simulink model "RobotX_TrajectoryPlanning"  (R2024a)
settings: Solver=ode45  StartTime=0.0  StopTime=17.77  MaxStep=1e-3  MinStep=1e-5  RelTol=1e-3
libraries: matrix_library x2, dspinverses x1, RobotX_Lib x1
settings Model: Creator=margaridaestrela  LastModifiedBy=margaridaestrela
settings SolverCC: MaxConsecutiveMinStep=100  ZeroCrossControl=DisableAll
settings DebuggingCC: SignalInfNanChecking=error

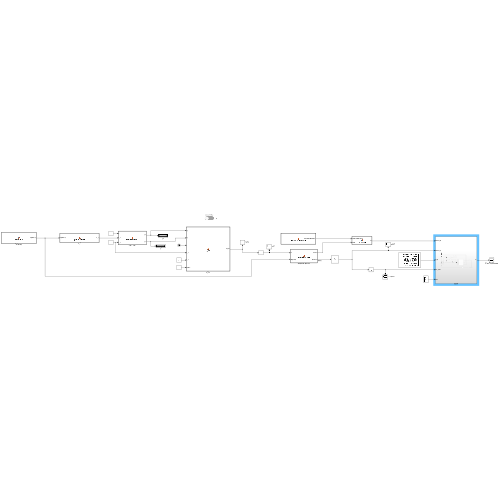
[thumbnail: Simulink's stored preview of the top-level diagram]
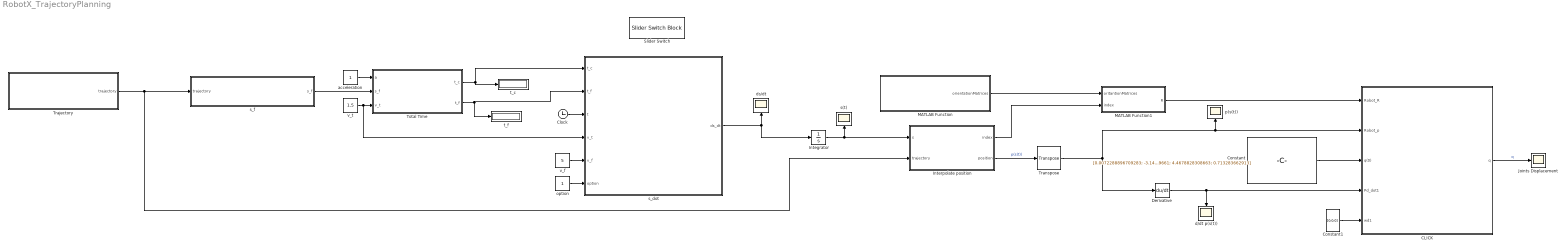
== system RobotX_TrajectoryPlanning ==
  CLICK : Subsystem
  Clock : Clock
  Constant : Constant  Value=[0.0072288896709283; -3.1404691212397; -57.815493873629; 68.626124143896; -3.1193903419661; 4.4678828308663; 0.713283662913]  VectorParams1D=off
  Constant1 : Constant  Value=[0;0;0]  VectorParams1D=off
  Derivative : Derivative
  Integrator : Integrator
  Interpolate position : MATLAB Function  TreatAsAtomicUnit=on
  Joints Displacement : Scope
  MATLAB Function : MATLAB Function  TreatAsAtomicUnit=on
  MATLAB Function1 : MATLAB Function  TreatAsAtomicUnit=on
  Slider Switch : SliderSwitchBlock
      settings: Values={{'1', '2'}, [1 2]}
  Total Time : MATLAB Function  TreatAsAtomicUnit=on
  Trajectory : MATLAB Function  TreatAsAtomicUnit=on
  Transpose : matrix_library/Transpose
  acceleration : Constant
  d/dt p(s(t)) : Scope
  ds/dt : Scope
  option : Constant
  p(s(t)) : Scope
  s(t) : Scope
  s_dot : MATLAB Function  TreatAsAtomicUnit=on
  s_f : MATLAB Function  TreatAsAtomicUnit=on
  t_c : Display
  t_f : Display
  v_f : Constant  Value=5
  v_t : Constant  Value=1.5
  wires:
  acceleration/1 -> Total Time/1(a)
  s_f/1(s_f) -> Total Time/2(s_f)
  Derivative/1 -> CLICK/4(Pd_dot1), d/dt p(s(t))/1
  v_t/1 -> s_dot/4(v_t), Total Time/3(v_t)
  Interpolate position/2(position) -> Transpose/1  "p(s(t))"
  Integrator/1 -> Interpolate position/1(s), s(t)/1
  s_dot/1(ds_dt) -> ds/dt/1, Integrator/1
  Total Time/1(t_c) -> s_dot/1(t_c), t_c/1
  Total Time/2(t_f) -> s_dot/2(t_f), t_f/1
  Trajectory/1(trajectory) -> Interpolate position/2(trajectory), s_f/1(trajectory)
  v_f/1 -> s_dot/5(v_f)
  option/1 -> s_dot/6(option)
  Transpose/1 -> Derivative/1, CLICK/2(Robot_p), p(s(t))/1
  Clock/1 -> s_dot/3(t)
  Constant/1 -> CLICK/3(q(0))
  MATLAB Function/1(orientationMatrices) -> MATLAB Function1/1(oritantionMatrices)
  Interpolate position/1(index) -> MATLAB Function1/2(index)
  Constant1/1 -> CLICK/5(wd1)
  MATLAB Function1/1(R) -> CLICK/1(Robot_R)
  CLICK/1(q) -> Joints Displacement/1  "q"

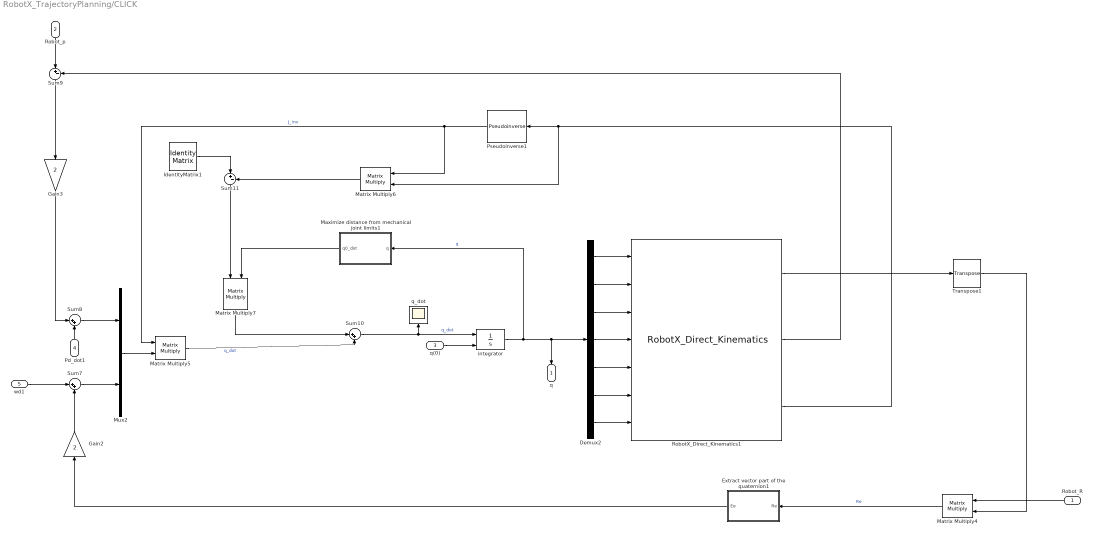
== system RobotX_TrajectoryPlanning/CLICK ==
  Robot_R : Inport
  Robot_p : Inport  Port=2
  q(0) : Inport  Port=3
  Pd_dot1 : Inport  Port=4
  wd1 : Inport  Port=5
  Demux2 : Demux  Outputs=7
  Extract vector part of the quaternion1 : MATLAB Function  TreatAsAtomicUnit=on
  Gain2 : Gain  Gain=2
  Gain3 : Gain  Gain=2
  IdentityMatrix1 : IdentityMatrix  OutputDimensions=7
  Matrix Multiply{4..7} (4 alike) : Product  Multiplication=Matrix(*)
  Maximize distance from mechanical joint limits1 : MATLAB Function  TreatAsAtomicUnit=on
  Mux2 : Mux  Inputs=2
  Pseudoinverse1 : dspinverses/Pseudoinverse  wanterr=off  SimulateUsing=Interpreted execution
  RobotX_Direct_Kinematics1 : RobotX_Lib/RobotX_Direct_Kinematics  SystemSampleTime=-1  VariantActivationTime=update diagram  AllowFlexibleInterface=on  Latency=0  AutoFrameSizeCalculation=off
  Sum10 : Sum  Inputs=|++
  Sum11 : Sum  Inputs=|+-
  Sum7 : Sum  Inputs=|++
  Sum8 : Sum  Inputs=|++
  Sum9 : Sum  Inputs=|+-
  Transpose1 : matrix_library/Transpose
  integrator : Integrator  InitialConditionSource=external
  q_dot : Scope
  q : Outport
  wires:
  Sum9/1 -> Gain3/1
  Matrix Multiply4/1 -> Extract vector part of the quaternion1/1(Re)  "Re"
  Matrix Multiply5/1 -> Sum10/2  "q_dot"
  Sum8/1 -> Mux2/1
  Robot_R/1 -> Matrix Multiply4/1
  Gain3/1 -> Sum8/1
  RobotX_Direct_Kinematics1/1 -> Transpose1/1
  integrator/1 -> q/1, Demux2/1, Maximize distance from mechanical joint limits1/1(q)  "q"
  Demux2/7 -> RobotX_Direct_Kinematics1/7
  RobotX_Direct_Kinematics1/3 -> Matrix Multiply6/2, Pseudoinverse1/1
  Maximize distance from mechanical joint limits1/1(q0_dot) -> Matrix Multiply7/2
  q(0)/1 -> integrator/2
  Gain2/1 -> Sum7/2
  Demux2/3 -> RobotX_Direct_Kinematics1/3
  Sum11/1 -> Matrix Multiply7/1
  Matrix Multiply6/1 -> Sum11/2
  Transpose1/1 -> Matrix Multiply4/2
  Demux2/4 -> RobotX_Direct_Kinematics1/4
  Demux2/5 -> RobotX_Direct_Kinematics1/5
  Demux2/6 -> RobotX_Direct_Kinematics1/6
  Pseudoinverse1/1 -> Matrix Multiply5/1, Matrix Multiply6/1  "J_inv"
  IdentityMatrix1/1 -> Sum11/1
  Mux2/1 -> Matrix Multiply5/2
  Robot_p/1 -> Sum9/1
  Sum7/1 -> Mux2/2
  Demux2/2 -> RobotX_Direct_Kinematics1/2
  Extract vector part of the quaternion1/1(Ee) -> Gain2/1
  Sum10/1 -> integrator/1, q_dot/1  "q_dot"
  RobotX_Direct_Kinematics1/2 -> Sum9/2
  Matrix Multiply7/1 -> Sum10/1
  Demux2/1 -> RobotX_Direct_Kinematics1/1
  wd1/1 -> Sum7/1
  Pd_dot1/1 -> Sum8/2

== matlab function RobotX_TrajectoryPlanning/Interpolate position ==
  data: index output; s input; trajectory input; position output
function [index, position] = interpolatePosition(s, trajectory)
    % Ensure s is within the bounds of cumulative distance
    cumulativeDistance = computeCumulativeDistance(trajectory);
    %s = min(max(s, cumulativeDistance(1)), cumulativeDistance(end));
    
    % Interpolate position
    position = interp1(cumulativeDistance, trajectory, s, 'linear', 'extrap');

    % Find the nearest index in the cumulative distance array
    [~, index] = min(abs(cumulativeDistance - s));
end

function cumulativeDistance = computeCumulativeDistance(trajectory)
    % Calculate distances between consecutive points
    distances = sqrt(sum(diff(trajectory).^2, 2));

    % Replace zeros with a small value (epsilon)
    eps = 1e-3;
    distances(distances == 0) = eps;
    
    % Calculate cumulative distance
    cumulativeDistance = [0; cumsum(distances)];
    
    % Ensure cumulativeDistance is strictly increasing by a minimum
    % difference of epsilon
    for i = 2:length(cumulativeDistance)
        while cumulativeDistance(i) <= cumulativeDistance(i-1) + eps;
            cumulativeDistance(i) = cumulativeDistance(i) + eps;
        end
    end
end

== matlab function RobotX_TrajectoryPlanning/CLICK/Extract vector part of the quaternion1 ==
  data: Re input; Ee output
function Ee = fcn(Re)
    % Initialize the output vector
    Ee = zeros(3, 1);

    % Compute the angle theta
    cos_theta = (Re(1,1) + Re(2,2) + Re(3,3) - 1) / 2;

    if cos_theta < -1 || cos_theta > 1
        return
    end

    theta = acos(cos_theta);

    % Initialize rx, ry, rz
    rx = 0;
    ry = 0;
    rz = 0;

    % Check for singularity at theta = 0 or theta = pi
    if sin(theta) == 0
        % Handle the case when theta is 0 or pi
        if cos_theta == 1
            % When theta is 0
            Ee = [0; 0; 0];
        else
            % When theta is pi
            % Choose the largest diagonal element for numerical stability
            [~, max_index] = max([Re(1,1), Re(2,2), Re(3,3)]);
            switch max_index
                case 1
                    rx = sqrt((Re(1,1) + 1) / 2);
                    ry = Re(2,1) / (2 * rx);
                    rz = Re(3,1) / (2 * rx);
                case 2
                    ry = sqrt((Re(2,2) + 1) / 2);
                    rx = Re(1,2) / (2 * ry);
                    rz = Re(3,2) / (2 * ry);
                case 3
                    rz = sqrt((Re(3,3) + 1) / 2);
                    rx = Re(1,3) / (2 * rz);
                    ry = Re(2,3) / (2 * rz);
            end
            Ee = [rx; ry; rz];
        end
    else
        % Compute the vector part for theta in (0, pi)
        rx = Re(3, 2) - Re(2, 3);
        ry = Re(1, 3) - Re(3, 1);
        rz = Re(2, 1) - Re(1, 2);
        Ee = (1 / (2 * sin(theta))) * [rx; ry; rz];
    end
end

== matlab function RobotX_TrajectoryPlanning/MATLAB Function ==
  data: orientationMatrices output
function orientationMatrices = loadOrientationMatrices
    data = load('orientationMatrices.mat');
    orientationMatrices = data.orientationMatrices;
end

== matlab function RobotX_TrajectoryPlanning/Trajectory ==
  data: trajectory output
function trajectory = loadTrajectory()
    data = load('trajectoryData.mat');
    trajectory = data.trajectory;
end

== matlab function RobotX_TrajectoryPlanning/s_f ==
  data: trajectory input; s_f output
function s_f = getTotalDistance(trajectory)
    distances = sqrt(sum(diff(trajectory).^2, 2));
    s_f = sum(distances);
end

== matlab function RobotX_TrajectoryPlanning/Total Time ==
  data: a input; s_f input; v_t input; t_c output; t_f output
function [t_c, t_f] = calculateTotalTime(a, s_f, v_t)
    % Calculate time to reach maximum velocity (acceleration phase)
    t_c = v_t / a;
    
    % Calculate distance covered during acceleration (and deceleration)
    d_c = 1/2 * a * t_c^2;
    
    % Calculate distance covered at constant velocity
    d_const = s_f - 2 * d_c;
    
    % Check if the distance for acceleration and deceleration is feasible
    if d_c * 2 > s_f
        error('Total distance is too short for the given acceleration and maximum velocity.');
    end
    
    % Calculate time for constant velocity phase
    t_const = d_const / v_t;
    
    % Total time of the trajectory
    t_f = t_c + t_const + t_c; % t_c is used for both acceleration and deceleration phases
end

== matlab function RobotX_TrajectoryPlanning/CLICK/Maximize distance from mechanical joint limits1 ==
  data: q0_dot output; q input
function q0_dot = fcn(q)
    n = length(q);  % Number of elements in q

    q_max = [350; deg2rad(170); deg2rad(45); deg2rad(156); deg2rad(185); deg2rad(120); deg2rad(350)];
    q_min = [-350; deg2rad(-170); deg2rad(-190); deg2rad(-120); deg2rad(-185); deg2rad(-120); deg2rad(-350)];

    q_dif = q_max - q_min;

    % Manually derive the differentiation
    w_diff = - (q - q_max) ./ (n * (q_dif.^2));
    
    q0_dot = 2 * w_diff;
end

== matlab function RobotX_TrajectoryPlanning/s_dot ==
  data: t_c input; t_f input; t input; v_t input; v_f input; ds_dt output; option input
function ds_dt = s_dot(t_c, t_f, t, v_t, v_f, option)
    if option == 1
        % Handle constant speed case
        ds_dt = zeros(size(t));
        for i = 1:length(t)
            if t(i) < 0
                ds_dt(i) = 0;
            elseif t(i) < t_c
                ds_dt(i) = (v_t / t_c) * t(i);
            elseif t(i) <= t_f - t_c
                ds_dt(i) = v_t;
            elseif t(i) <= t_f
                ds_dt(i) = v_t - (v_t / t_c) * (t(i) - (t_f - t_c));
            else
                ds_dt(i) = 0;
            end
        end
    else
        % Handle feed velocity case
        ds_dt = zeros(size(t));
        for i = 1:length(t)
            if t(i) < 0
                ds_dt(i) = 0;
            elseif t(i) < t_c
                ds_dt(i) = (v_f / t_c) * t(i);
            elseif t(i) <= t_f - t_c
                ds_dt(i) = v_f;
            elseif t(i) <= t_f
                ds_dt(i) = v_f - (v_f / t_c) * (t(i) - (t_f - t_c));
            else
                ds_dt(i) = 0;
            end
        end
    end
end

== matlab function RobotX_TrajectoryPlanning/MATLAB Function1 ==
  data: oritantionMatrices input; index input; R output
function R = getRotation(oritantionMatrices, index)
    R = oritantionMatrices(:, :, index);
end
